simulink model "TopLevelModel"  (R2023a)
settings: Solver=VariableStepAuto  StartTime=0.0  StopTime=inf  RelTol=1e-3
values from neighbouring files (symbols this model uses):
  b = 40.6518    [TopLevelModelParameters.m]
  B1 = 0.0042    [TopLevelModelParameters.m]
  B2 = 0.0084    [TopLevelModelParameters.m]
  J1 = 7e-5    (= 7e-05)    [TopLevelModelParameters.m]
  J2 = 8e-5    (= 8e-05)    [TopLevelModelParameters.m]
  k1 = 2.6552e5    (= 265520)    [TopLevelModelParameters.m]
  k2 = 2.6552e5    (= 265520)    [TopLevelModelParameters.m]
  k3 = 11.777e4    (= 117770)    [TopLevelModelParameters.m]
  Kb = 23e-3    (= 0.023)    [TopLevelModelParameters.m]
  Kt = 23e-3    (= 0.023)    [TopLevelModelParameters.m]
  L = 0.1    [TopLevelModelParameters.m]
  m = 2    [TopLevelModelParameters.m]
  R = 0.71    [TopLevelModelParameters.m]
  r = 0.0194    [TopLevelModelParameters.m]
undefined symbols (not defined in the file or in its folder): J, Kd, Ke
libraries: fl_lib x40, fl_ps_legacy_lib x16, nesl_utility x12, slpidlib x10, SignalEditorBlockLib x4, ee_lib x4, simulink x2
(part 1 of 3)
settings Model: PacingRate=10  Creator=M3tal  LastModifiedBy=M3tal
settings OptimizationCC: DefaultParameterBehavior=Inlined  EnhancedBackFolding=on  PassReuseOutputArgsThreshold=0  OptimizeBlockOrder=speed  DifferentSizesBufferReuse=on
settings DebuggingCC: ParameterTunabilityLossMsg=error
settings HardwareCC: TargetBitPerPointer=64  TargetBitPerSizeT=64  TargetBitPerPtrDiffT=64  TargetLongLongMode=on  TargetIntDivRoundTo=Zero  TargetEndianess=LittleEndian  TargetWordSize=64  TargetHWDeviceType=MATLAB Host  ProdEqTarget=off
settings SFSimCC: MATLABDynamicMemAlloc=off
settings RTWCC: GenCodeOnly=on
settings CodeAppCC: ForceParamTrailComments=on  OperatorAnnotations=on
settings ConfigComp: PLC_TargetIDE=codesys23  PLC_MultiTBSigbuilderTimeRange=off  PLC_FoldFBCallOutputVar=off  PLC_RemoveUnusedSSMethodCallArguments=off  PLC_UseCallOutputArgSyntax=off  PLC_EnableUnsignedAndDoubleTypes=off  PLC_EnableUDTSplitting=off  PLC_MaxFieldsInUDT=500  PLC_InlineEnumCastFunction=off

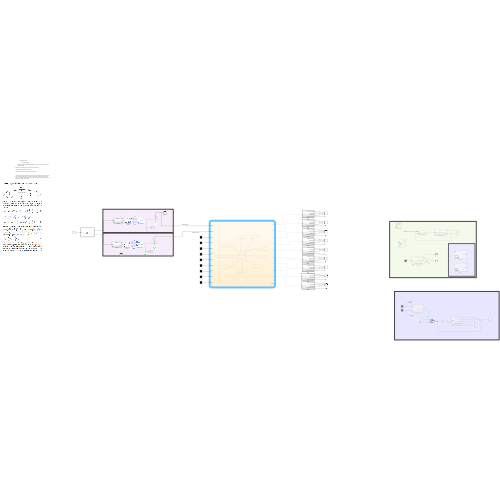
[thumbnail: Simulink's stored preview of the top-level diagram]
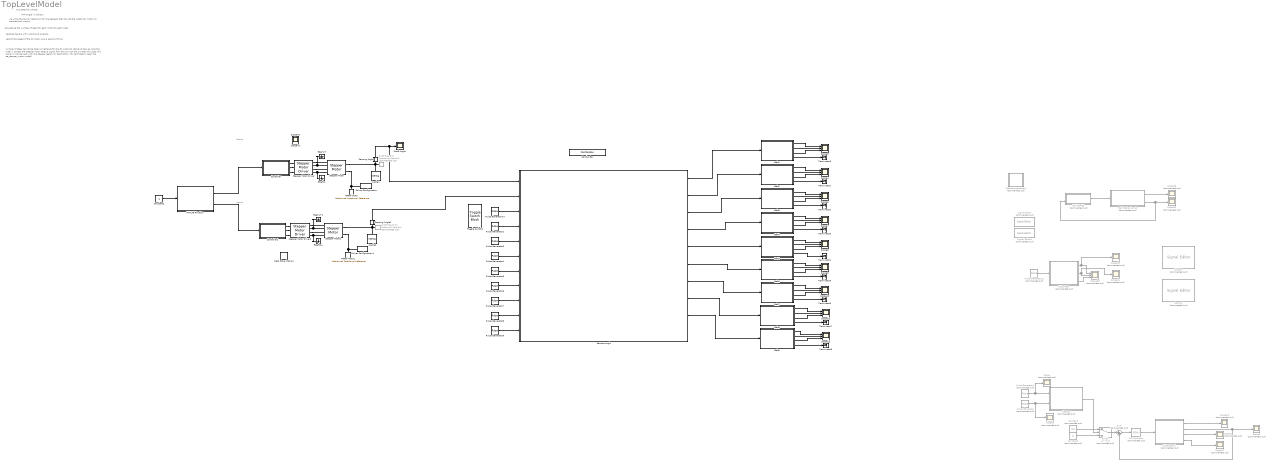
== system TopLevelModel ==
  note: two state flow charts
  note: number of steps cannot be taken as refrence for the dc motors to start and stop as once the meal is chosen the stepper motor takes a signal from the plc with the number of pulses, this signal is maintained unitll the stepper reachs it's destination. (for calrification open the ee_stepper_motor model)
  note: X-axis
  note: -replace signals with inports and outports
  note: -record the speed of the dc motor over a period of time
  note: -caluclating the number of steps for each motor for each meal
  note: Y-axis
  note: we using the same mechansim for the steppers that convert the rotational motion to translational motion
  note: m=r*angle in radians
  Belt Mechanism10 : Subsystem  Commented=on
  Belt1 : Subsystem  TreatAsAtomicUnit=on
  Belt2 : Subsystem  TreatAsAtomicUnit=on
  Belt3 : Subsystem  TreatAsAtomicUnit=on
  Belt4 : Subsystem  TreatAsAtomicUnit=on
  Belt5 : Subsystem  TreatAsAtomicUnit=on
  Belt6 : Subsystem  TreatAsAtomicUnit=on
  Belt7 : Subsystem  TreatAsAtomicUnit=on
  Belt8 : Subsystem  TreatAsAtomicUnit=on
  Belt9 : Subsystem  TreatAsAtomicUnit=on
  Combo Box : ComboBox  LabelPosition=Hide  SelectedLabel=1
      settings: Values={{'1', '2', '3', '4', '5', '6', '7', '8', '9', '0'}, [1 2 3 4 5 6 7 8 9 0]}
  Constant : Constant  Commented=on  Value=0.2
  Constant1 : Constant  Commented=on  Value=0
  Constant2 : Constant
  Controller : Subsystem  Variant=on  VariantControlMode=label  LabelModeActiveChoice=Position
      settings: AttributesFormatString=%<BlockChoice>
  Controller1 : Subsystem  Variant=on  VariantControlMode=label  LabelModeActiveChoice=Position
      settings: AttributesFormatString=%<BlockChoice>
  DC Motor10 : Subsystem  Commented=on
  Data Store Memory : DataStoreMemory  DataStoreName=counter  WriteAfterWriteMsg=warning  ShowAdditionalParam=off
  ERef A+ : fl_lib/Electrical/Electrical Elements/Electrical Reference
  ERef A+1 : fl_lib/Electrical/Electrical Elements/Electrical Reference
  ERef B- : fl_lib/Electrical/Electrical Elements/Electrical Reference
  ERef B-1 : fl_lib/Electrical/Electrical Elements/Electrical Reference
  Inertia1 : fl_lib/Mechanical/Rotational Elements/Inertia  inertia=0.1 kg*m^2  num_ports=foundation.enum.numPorts2.one  w_specify=off  w_priority=High  w=0 rad/s  w_nominal_specify=off  w_nominal_unit=rad/s  w_nominal_value=1  t_specify=off  t_priority=None  t=0 N*m  t_nominal_specify=off  t_nominal_unit=N*m  t_nominal_value=1
  Inertia2 : fl_lib/Mechanical/Rotational Elements/Inertia  inertia=0.1 kg*m^2  num_ports=foundation.enum.numPorts2.one  w_specify=off  w_priority=High  w=0 rad/s  w_nominal_specify=off  w_nominal_unit=rad/s  w_nominal_value=1  t_specify=off  t_priority=None  t=0 N*m  t_nominal_specify=off  t_nominal_unit=N*m  t_nominal_value=1
  MATLAB Function : MATLAB Function  TreatAsAtomicUnit=on
  MRRef Motor : fl_lib/Mechanical/Rotational Elements/Mechanical Rotational Reference
  MRRef Motor1 : fl_lib/Mechanical/Rotational Elements/Mechanical Rotational Reference
  PID Controller : slpidlib/PID Controller  Commented=on  Controller=PID  Form=Parallel  TimeDomain=Continuous-time  UseExternalTs=off  SampleTime=-1  IntegratorMethod=Forward Euler  FilterMethod=Forward Euler  ControllerParametersSource=internal  P=29.8496571480823  I=152.933850283855  UseKiTs=off  D=-0.451147774638306  N=4.48716691500189  UseFilter=on  TunerSelectOption=Transfer Function Based (PID Tuner App)  InitialConditionSource=internal  InitialConditionForIntegrator=0  InitialConditionForFilter=0  DifferentiatorICPrevScaledInput=0  ExternalReset=none  TrackingMode=off  Kt=1  LimitOutput=off  SatLimitsSource=internal  UpperSaturationLimit=inf  LowerSaturationLimit=-inf  LinearizeAsGain=on  AntiWindupMode=none  Kb=1  LimitIntegrator=off  UpperIntegratorSaturationLimit=inf  LowerIntegratorSaturationLimit=-inf  POutMin=[]  POutMax=[]  IOutMin=[]  IOutMax=[]  DOutMin=[]  DOutMax=[]  NOutMin=[]  NOutMax=[]  SumOutMin=[]  SumOutMax=[]  SaturationOutMin=[]  SaturationOutMax=[]  PParamMin=[]  PParamMax=[]  IParamMin=[]  IParamMax=[]  DParamMin=[]  DParamMax=[]  NParamMin=[]  NParamMax=[]  KbParamMin=[]  KbParamMax=[]  KtParamMin=[]  KtParamMax=[]  KbOutMin=[]  KbOutMax=[]  KtOutMin=[]  KtOutMax=[]  IntegratorOutMin=[]  IntegratorOutMax=[]  FilterOutMin=[]  FilterOutMax=[]  SumI1OutMin=[]  SumI1OutMax=[]  SumI2OutMin=[]  SumI2OutMax=[]  SumI3OutMin=[]  SumI3OutMax=[]  SumI4OutMin=[]  SumI4OutMax=[]  SumDOutMin=[]  SumDOutMax=[]  DifferentiatorOutMin=[]  DifferentiatorOutMax=[]  FilterDiffOutCoefMin=[]  FilterDiffOutCoefMax=[]  ReciprocalOutMin=[]  ReciprocalOutMax=[]  SumDenOutMin=[]  SumDenOutMax=[]  SumNumOutMin=[]  SumNumOutMax=[]  DivideOutMin=[]  DivideOutMax=[]  UdiffTsProdOutMin=[]  UdiffTsProdOutMax=[]  NTsProdOutMin=[]  NTsProdOutMax=[]  UintegralTsProdOutMin=[]  UintegralTsProdOutMax=[]  UngainTsProdOutMin=[]  UngainTsProdOutMax=[]  ClampingZeroOutDataTypeStr=Inherit: Inherit via back propagation  ClampingZeroOutMin=[]  ClampingZeroOutMax=[]  FilterDenConstantOutDataTypeStr=Inherit: Inherit via back propagation  FilterDenConstantOutMin=[]  FilterDenConstantOutMax=[]  PCopyOutDataTypeStr=Inherit: Inherit via back propagation  PCopyOutMin=[]  PCopyOutMax=[]  NCopyOutDataTypeStr=Inherit: Inherit via back propagation  NCopyOutMin=[]  NCopyOutMax=[]  IntegratorContinuousStateAttributes=''  IntegratorStateMustResolveToSignalObject=off  IntegratorRTWStateStorageClass=Auto  FilterContinuousStateAttributes=''  FilterStateMustResolveToSignalObject=off  FilterRTWStateStorageClass=Auto  ParallelPVariant=InternalParameters  IdealPVariant=Disabled  IVariant=InternalParameters  DVariant=InternalParameters  IntegratorVariant=Continuous  SatVariant=Disabled  AWVariant=Passthrough  PCopyVariant=Disabled  TRVariant=Disabled  FdbkBlocksVariant=Forward  IdealPFdbkVariant=Disabled  SatFdbkVariant=Disabled  DerivativeFilterVariant=ContFilter  NVariant=InternalParameters  NCopyVariant=Disabled  FilterICVariant=InternalICsFilter  IntegratorICVariant=InternalICs  ExternalResetVariant=Disabled  TRSumVariant=Passthrough  SumFdbkVariant=Disabled  SumVariant=Sum_PID  TsampFilterVariant=InternalTs  TsampNgainVariant=Passthrough  TsampIntegralVariant=Disabled_SignalSpec  ExternalSaturationOutDataTypeStr=Inherit: Same as second input
  Pulse Generator : DiscretePulseGenerator  Commented=on  PulseType=Time based  Period=40  PhaseDelay=20
  Pulse Generator1 : DiscretePulseGenerator  Commented=on  PulseType=Time based  Period=50  PhaseDelay=5
  Pulse Generator11 : DiscretePulseGenerator  Commented=on  PulseType=Time based  Amplitude=12  Period=11  PulseWidth=50  PhaseDelay=2
  Pulse Generator14 : DiscretePulseGenerator  PulseType=Time based  Period=10  PulseWidth=5
  Pulse Generator{2..9} (8 alike) : DiscretePulseGenerator  PulseType=Time based  Amplitude=0  Period=10  PulseWidth=5
  Scope{,1..3,24..29} (10 alike) : Scope  Commented=on
  Scope{4..12} (9 alike) : Scope  NumInputPorts=3
  Scope23 : Scope  Commented=on  NumInputPorts=3
  Sensing Angle : Subsystem
      mask Display: disp('a')
  Sensing Angle1 : Subsystem
      mask Display: disp('a')
  Sensor : SignalEditorBlockLib/Signal Editor  Commented=on  FileName=Crane_Sensor.mat  ActiveScenario=Scenario  ActiveSignal=Crane signal  IsBus=off  OutputBusObjectStr=Bus: BusObject  SampleTime=0  Interpolate=off  ZeroCross=off  OutputAfterFinalValue=Setting to zero  Unit=inherit  PreserveSignalName=on  ApplySigPropsToAllScenarios=on
  Sensor1 : SignalEditorBlockLib/Signal Editor  Commented=on  FileName=Belt_Sensor.mat  ActiveScenario=Scenario  ActiveSignal=Belt Signal  IsBus=off  OutputBusObjectStr=Bus: BusObject  SampleTime=0  Interpolate=off  ZeroCross=off  OutputAfterFinalValue=Setting to zero  Unit=inherit  PreserveSignalName=on  ApplySigPropsToAllScenarios=on
  Sensors : Stateflow chart  Commented=on  TreatAsAtomicUnit=on
  Sensors Logic : Stateflow chart  TreatAsAtomicUnit=on
      settings: PortSchema="{\"entries\":[{\"content\":{\"sides\":[{\"content\":{\"connectorIds\":[\"In10\",\"In11\",\"In1\",\"In2\",\"In3\",\"In4\",\"In5\",\"In6\",\"In7\",\"In8\",\"In9\"]},\"type\":\"ConnectorPlacement.EquallySpacedRectSide\",\"uuid\":\"dd9ce701-3689-4654-9b21-5529dab0541a\"},{\"content\":{\"connectorIds\":[\"Out1\",\"Out2\",\"Out3\",\"Out4\",\"Out5\",\"Out6\",\"Out7\",\"Out8\",\"Out9\",\"Out10\"],\"side\":\"RIGHT\"},\"type\":\"ConnectorPlacement.EquallySpacedRectSide\",\"uuid\":\"ff8f0f67-846c-4703-aeda-d87216d47c92\"},{\"content\":{\"side\":\"TOP\"},\"type\":\"ConnectorPlacement.EquallySpacedRectSide\",\"uuid\":\"ae968bb7-da0f-44fd-802b-06f57922bbce\"},{\"content\":{\"side\":\"BOTTOM\"},\"type\":\"ConnectorPlacement.EquallySpacedRectSide\",\"uuid\":\"72f2caf6-56e4-41be-9339-a06e52f77ea7\"}]},\"type\":\"ConnectorPlacement.EquallySpacedConnector\",\"uuid\":\"820653e5-881f-4b8b-9810-894dc5dde637\"}],\"packageUris\":[\"http://schema.mathworks.com/mf0/Connector/R2020b\"],\"version\":\"1.0\"}"
  Shaft Angle : Scope
  Shaft Free End : fl_lib/Mechanical/Rotational Elements/Rotational Free End  Commented=on  w_specify=off  w_priority=None  w=0 rad/s  w_nominal_specify=off  w_nominal_unit=rad/s  w_nominal_value=1
  Shaft Free End1 : fl_lib/Mechanical/Rotational Elements/Rotational Free End  Commented=on  w_specify=off  w_priority=None  w=0 rad/s  w_nominal_specify=off  w_nominal_unit=rad/s  w_nominal_value=1
  Signal Editor : SignalEditorBlockLib/Signal Editor  Commented=on  FileName=X_Position.mat  ActiveScenario=Scenario  ActiveSignal=X  IsBus=off  OutputBusObjectStr=Bus: BusObject  SampleTime=0  Interpolate=off  ZeroCross=off  OutputAfterFinalValue=Setting to zero  Unit=inherit  PreserveSignalName=on  ApplySigPropsToAllScenarios=on
  Signal Editor1 : SignalEditorBlockLib/Signal Editor  Commented=on  FileName=Y_Position.mat  ActiveScenario=Scenario  ActiveSignal=Y  IsBus=off  OutputBusObjectStr=Bus: BusObject  SampleTime=0  Interpolate=off  ZeroCross=off  OutputAfterFinalValue=Setting to zero  Unit=inherit  PreserveSignalName=on  ApplySigPropsToAllScenarios=on
  Solver Configuration : nesl_utility/Solver Configuration  PhysicalDomain=network_engine_domain  SubClassName=solver  LeftPortType=input  RightPortType=generic  Tones=[]  Harmonics=[]  SimulateNoise=off  Profile=off  UseLocalSampling=off  EnableSwitchedLinearOptims=on  FrequencyDomain=off  UseCCode=off  RelTol=0.001  AbsTol=1e-06  MinStep=1e-09  ToWorkspace=off  RevertToSquareIcSolve=off  NumHomotopyIterations=100  PhasorMode=off  PhasorModeNumHarmonics=1  ConsistencySolver=NEWTON_FTOL  IndexReductionMethod=DerivativeReplacement  DoDC=off  ResidualTolerance=1e-9  ConsistencyTolSource=GLOBAL  ConsistencyAbsTol=0.001  ConsistencyRelTol=0.001  ConsistencyTolFactor=0.001  UseLocalSolver=off  LocalSolverChoice=NE_BACKWARD_EULER_ADVANCER  ResolveIndetEquations=on  FunctionEvalNumThread=1  LocalSolverSampleTime=.001  DoFixedCost=off  MaxNonlinIter=3  MaxModeIter=2  ComputeImpulses=off  ImpulseIterations=2  LinearAlgebra=auto  LinearAlgebraNumThread=0  EquationFormulation=NE_TIME_EF  DelaysMemoryBudget=1024  AutomaticFiltering=on  FilteringTimeConstant=0.001  PartitionStorageMethod=AS_NEEDED  PartitionMemoryBudget=1024  PartitionMethod=FAST
  Solver Configuration1 : nesl_utility/Solver Configuration  PhysicalDomain=network_engine_domain  SubClassName=solver  LeftPortType=input  RightPortType=generic  Tones=[]  Harmonics=[]  SimulateNoise=off  Profile=off  UseLocalSampling=off  EnableSwitchedLinearOptims=on  FrequencyDomain=off  UseCCode=off  RelTol=0.001  AbsTol=1e-06  MinStep=1e-09  ToWorkspace=off  RevertToSquareIcSolve=off  NumHomotopyIterations=100  PhasorMode=off  PhasorModeNumHarmonics=1  ConsistencySolver=NEWTON_FTOL  IndexReductionMethod=DerivativeReplacement  DoDC=off  ResidualTolerance=1e-9  ConsistencyTolSource=GLOBAL  ConsistencyAbsTol=0.001  ConsistencyRelTol=0.001  ConsistencyTolFactor=0.001  UseLocalSolver=off  LocalSolverChoice=NE_BACKWARD_EULER_ADVANCER  ResolveIndetEquations=on  FunctionEvalNumThread=1  LocalSolverSampleTime=.001  DoFixedCost=off  MaxNonlinIter=3  MaxModeIter=2  ComputeImpulses=off  ImpulseIterations=2  LinearAlgebra=auto  LinearAlgebraNumThread=0  EquationFormulation=NE_TIME_EF  DelaysMemoryBudget=1024  AutomaticFiltering=on  FilteringTimeConstant=0.001  PartitionStorageMethod=AS_NEEDED  PartitionMemoryBudget=1024  PartitionMethod=FAST
  Stepper Motor : ee_lib/Electromechanical/Reluctance & Stepper/Stepper Motor  step_or_av=ee.enum.electromech.simulationMode.stepping  Ra=1.3 Ohm  La=2.9 mH  Km=0.315 N*m/A  Td=25 mN*m  Rm=Inf Ohm  w_vec=[ 0 1000 3e+3 ] rpm  T_vec=[ 2 2 1 ] N*m  assert_if_slipping=0  J_total=1e-4 kg*m^2  max_step_rate=10 Hz  Step=1.8 deg  J=82 g*cm^2  B=1e-2 N*m/(rad/s)  speed0=0 rpm  theta0=0 deg  alpha=[.00393, .00393] 1/K  Tmeas=25 degC  Tmeas2=125 degC  T_vec2=[1.7, 1.7, .85] N*m  half_stepping=ee.enum.electromech.steppingModeAveraged.fullStep  thermal_masses=[100, 100] J/K  initial_temperatures=[25, 25] degC  rotor_thermal_mass=50 J/K  rotor_initial_temperature=25 degC  Rm_percent_rotor=90
      settings: InternalSimscapePortConfiguration="{\"Bottom\":[],\"Left\":[{\"id\":\"pA\",\"label\":\"A+\",\"type\":\"foundation.electrical.electrical\"},{\"id\":\"nA\",\"label\":\"A-\",\"type\":\"foundation.electrical.electrical\"},{\"id\":\"pB\",\"label\":\"B+\",\"type\":\"foundation.electrical.electrical\"},{\"id\":\"nB\",\"label\":\"B-\",\"type\":\"foundation.electrical.electrical\"}],\"Right\":[{\"id\":\"R\",\"label\":\"R\",\"type\":\"foundation.mechanical.rotational.rotational\"},{\"id\":\"C\",\"label\":\"C\",\"type\":\"foundation.mechanical.rotational.rotational\"}],\"Top\":[]}"
  Stepper Motor Driver : ee_lib/Electromechanical/Reluctance & Stepper/Stepper Motor Driver  step_or_av=1  step_rate_per_volt=10 Hz/V  Venable=2.5 V  Vreverse=2.5 V  supply_ports=ee.enum.supply_ports.hidesupply  Vm=5 V  Vsupply=10 V  half_stepping=0  stepping_mode=ee.enum.electromech.steppingMode.fullStep  numMicroSteps=4  Im=1.2 A
      settings: InternalSimscapePortConfiguration="{\"Bottom\":[],\"Left\":[{\"id\":\"ENA\",\"label\":\"ENA\",\"type\":\"foundation.electrical.electrical\"},{\"id\":\"REF\",\"label\":\"REF\",\"type\":\"foundation.electrical.electrical\"},{\"id\":\"REV\",\"label\":\"REV\",\"type\":\"foundation.electrical.electrical\"}],\"Right\":[{\"id\":\"pA\",\"label\":\"A+\",\"type\":\"foundation.electrical.electrical\"},{\"id\":\"nA\",\"label\":\"A-\",\"type\":\"foundation.electrical.electrical\"},{\"id\":\"pB\",\"label\":\"B+\",\"type\":\"foundation.electrical.electrical\"},{\"id\":\"nB\",\"label\":\"B-\",\"type\":\"foundation.electrical.electrical\"}],\"Top\":[]}"
  Stepper Motor Driver1 : ee_lib/Electromechanical/Reluctance & Stepper/Stepper Motor Driver  step_or_av=1  step_rate_per_volt=10 Hz/V  Venable=2.5 V  Vreverse=2.5 V  supply_ports=ee.enum.supply_ports.hidesupply  Vm=5 V  Vsupply=10 V  half_stepping=0  stepping_mode=ee.enum.electromech.steppingMode.fullStep  numMicroSteps=4  Im=1.2 A
      settings: InternalSimscapePortConfiguration="{\"Bottom\":[],\"Left\":[{\"id\":\"ENA\",\"label\":\"ENA\",\"type\":\"foundation.electrical.electrical\"},{\"id\":\"REF\",\"label\":\"REF\",\"type\":\"foundation.electrical.electrical\"},{\"id\":\"REV\",\"label\":\"REV\",\"type\":\"foundation.electrical.electrical\"}],\"Right\":[{\"id\":\"pA\",\"label\":\"A+\",\"type\":\"foundation.electrical.electrical\"},{\"id\":\"nA\",\"label\":\"A-\",\"type\":\"foundation.electrical.electrical\"},{\"id\":\"pB\",\"label\":\"B+\",\"type\":\"foundation.electrical.electrical\"},{\"id\":\"nB\",\"label\":\"B-\",\"type\":\"foundation.electrical.electrical\"}],\"Top\":[]}"
  Stepper Motor1 : ee_lib/Electromechanical/Reluctance & Stepper/Stepper Motor  step_or_av=ee.enum.electromech.simulationMode.stepping  Ra=1.3 Ohm  La=2.9 mH  Km=0.315 N*m/A  Td=25 mN*m  Rm=Inf Ohm  w_vec=[ 0 1000 3e+3 ] rpm  T_vec=[ 2 2 1 ] N*m  assert_if_slipping=0  J_total=1e-4 kg*m^2  max_step_rate=10 Hz  Step=1.8 deg  J=82 g*cm^2  B=1e-2 N*m/(rad/s)  speed0=0 rpm  theta0=0 deg  alpha=[.00393, .00393] 1/K  Tmeas=25 degC  Tmeas2=125 degC  T_vec2=[1.7, 1.7, .85] N*m  half_stepping=ee.enum.electromech.steppingModeAveraged.fullStep  thermal_masses=[100, 100] J/K  initial_temperatures=[25, 25] degC  rotor_thermal_mass=50 J/K  rotor_initial_temperature=25 degC  Rm_percent_rotor=90
      settings: InternalSimscapePortConfiguration="{\"Bottom\":[],\"Left\":[{\"id\":\"pA\",\"label\":\"A+\",\"type\":\"foundation.electrical.electrical\"},{\"id\":\"nA\",\"label\":\"A-\",\"type\":\"foundation.electrical.electrical\"},{\"id\":\"pB\",\"label\":\"B+\",\"type\":\"foundation.electrical.electrical\"},{\"id\":\"nB\",\"label\":\"B-\",\"type\":\"foundation.electrical.electrical\"}],\"Right\":[{\"id\":\"R\",\"label\":\"R\",\"type\":\"foundation.mechanical.rotational.rotational\"},{\"id\":\"C\",\"label\":\"C\",\"type\":\"foundation.mechanical.rotational.rotational\"}],\"Top\":[]}"
  SteppermotorsLogic : Stateflow chart  Commented=on  TreatAsAtomicUnit=on
  Subsystem : Subsystem  Commented=on
  Subsystem1 : Subsystem  Commented=on
  Sum : Sum  Commented=on  Inputs=|+-
  Switch : Switch  Commented=on  Criteria=u2 ~= 0  Threshold=1  SaturateOnIntegerOverflow=off  InputSameDT=off
  Terminator{1..9} (9 alike) : Terminator
  Toggle Switch2 : ToggleSwitchBlock
      settings: Values={{'Off', 'On'}, [0 1]}
  Scope41 : Scope
  Scope42 : Scope
  wires:
  Pulse Generator1/1 -> Scope/1, Sensors/1(Crane)
  Subsystem1/2(load velocity) -> Sum/2, Scope2/1  "Velocity"
  Pulse Generator/1 -> Scope3/1, Sensors/2(Belt)
  Subsystem/1(drive pulley velocity) -> Scope25/1, Scope23/1
  Subsystem/2(load velocity) -> Scope23/2, Scope24/1
  Subsystem/3(driven pulley velocity) -> Scope23/3
  Pulse Generator11/1 -> Subsystem/1(Voltage)
  Sum/1 -> PID Controller/1
  Sensors/1(Voltage) -> Switch/2
  Constant1/1 -> Switch/3
  PID Controller/1 -> Subsystem1/1(Voltage)
  Switch/1 -> Sum/1
  Constant/1 -> Switch/1
  Subsystem1/1(drive pulley velocity) -> Scope26/1
  Subsystem1/4(driven pulley Velocity) -> Scope27/1
  Subsystem1/3(load position) -> Scope1/1
  Constant2/1 -> MATLAB Function/1(meal)
  ? -> DC Motor10/1(Voltage)
  Belt Mechanism10/2(Velocity) -> Scope29/1, DC Motor10/2(Velocity)  "Velocity"
  Belt Mechanism10/1(Position) -> Scope28/1
  DC Motor10/1(Tourque) -> Belt Mechanism10/1(Tourque)  "Tourque"
  Sensing Angle/1(theta) -> Sensors Logic/10(XTheta), Shaft Angle/1  "XTheta (degrees)"
  Sensing Angle1/1(theta) -> Sensors Logic/11(YTheta)  "YTheta (degrees)"
  MATLAB Function/1(x) -> Controller/1(Ref)
  Pulse Generator14/1 -> Sensors Logic/1(Belt1)
  MATLAB Function/2(y) -> Controller1/1(Ref)
  Sensors Logic/1(V1) -> Belt1/1(V1)
  Belt1/4(driven pulley Velocity) -> Terminator9/1
  Belt1/1(drive pulley velocity) -> Scope5/1
  Belt1/2(load velocity) -> Scope5/2
  Belt1/3(load position) -> Scope5/3
  Belt2/1(drive pulley velocity) -> Scope4/1
  Belt2/3(load position) -> Scope4/3
  Belt2/4(driven pulley Velocity) -> Terminator1/1
  Belt2/2(load velocity) -> Scope4/2
  Sensors Logic/2(V2) -> Belt2/1(V1)
  Belt3/2(load velocity) -> Scope6/2
  Belt3/1(drive pulley velocity) -> Scope6/1
  Belt3/3(load position) -> Scope6/3
  Belt3/4(driven pulley Velocity) -> Terminator2/1
  Sensors Logic/3(V3) -> Belt3/1(V1)
  Belt4/4(driven pulley Velocity) -> Terminator3/1
  Belt4/3(load position) -> Scope7/3
  Belt4/2(load velocity) -> Scope7/2
  Belt4/1(drive pulley velocity) -> Scope7/1
  Sensors Logic/4(V4) -> Belt4/1(V1)
  Sensors Logic/5(V5) -> Belt5/1(V1)
  Belt5/3(load position) -> Scope8/3
  Belt5/1(drive pulley velocity) -> Scope8/1
  Belt5/4(driven pulley Velocity) -> Terminator4/1
  Belt5/2(load velocity) -> Scope8/2
  Belt6/2(load velocity) -> Scope9/2
  Belt6/4(driven pulley Velocity) -> Terminator5/1
  Belt6/3(load position) -> Scope9/3
  Belt6/1(drive pulley velocity) -> Scope9/1
  Sensors Logic/6(V6) -> Belt6/1(V1)
  Belt7/3(load position) -> Scope10/3
  Belt7/1(drive pulley velocity) -> Scope10/1
  Belt7/2(load velocity) -> Scope10/2
  Belt7/4(driven pulley Velocity) -> Terminator6/1
  Sensors Logic/7(V7) -> Belt7/1(V1)
  Belt8/1(drive pulley velocity) -> Scope11/1
  Belt8/3(load position) -> Scope11/3
  Belt8/4(driven pulley Velocity) -> Terminator7/1
  Belt8/2(load velocity) -> Scope11/2
  Sensors Logic/8(V8) -> Belt8/1(V1)
  Belt9/3(load position) -> Scope12/3
  Belt9/2(load velocity) -> Scope12/2
  Belt9/4(driven pulley Velocity) -> Terminator8/1
  Belt9/1(drive pulley velocity) -> Scope12/1
  Sensors Logic/9(V9) -> Belt9/1(V1)
  Pulse Generator2/1 -> Sensors Logic/2(Belt2)
  Pulse Generator4/1 -> Sensors Logic/4(Belt4)
  Pulse Generator3/1 -> Sensors Logic/3(Belt3)
  Pulse Generator5/1 -> Sensors Logic/5(Belt5)
  Pulse Generator6/1 -> Sensors Logic/6(Belt6)
  Pulse Generator7/1 -> Sensors Logic/7(Belt7)
  Pulse Generator8/1 -> Sensors Logic/8(Belt8)
  Pulse Generator9/1 -> Sensors Logic/9(Belt9)
  connections:
  MRRef Motor/LConn1 -- Stepper Motor/RConn2 -- Solver Configuration/RConn1
  Stepper Motor/LConn4 -- Stepper Motor Driver/RConn4 -- ERef B-/LConn1
  Stepper Motor Driver/RConn2 -- Stepper Motor/LConn2 -- ERef A+/LConn1
  Sensing Angle/LConn1 -- Stepper Motor/RConn1 -- Inertia1/LConn1 -- Shaft Free End/LConn1
  Stepper Motor Driver/RConn1 -- Stepper Motor/LConn1
  Controller/RConn2 -- Stepper Motor Driver/LConn2
  Controller/RConn3 -- Stepper Motor Driver/LConn3
  Controller/RConn1 -- Stepper Motor Driver/LConn1
  Stepper Motor Driver/RConn3 -- Stepper Motor/LConn3
  ERef B-1/LConn1 -- Stepper Motor1/LConn4 -- Stepper Motor Driver1/RConn4
  Solver Configuration1/RConn1 -- MRRef Motor1/LConn1 -- Stepper Motor1/RConn2
  ERef A+1/LConn1 -- Stepper Motor Driver1/RConn2 -- Stepper Motor1/LConn2
  Sensing Angle1/LConn1 -- Stepper Motor1/RConn1 -- Inertia2/LConn1 -- Shaft Free End1/LConn1
  Controller1/RConn3 -- Stepper Motor Driver1/LConn3
  Controller1/RConn1 -- Stepper Motor Driver1/LConn1
  Stepper Motor Driver1/RConn1 -- Stepper Motor1/LConn1
  Stepper Motor Driver1/RConn3 -- Stepper Motor1/LConn3
  Controller1/RConn2 -- Stepper Motor Driver1/LConn2

== system TopLevelModel/Belt Mechanism10 ==
  note: Note: The term $K \frac{d\theta}{dt}$ ​ represents a damping torque that is proportional to the angular velocity
  note: $\frac{d^2\theta}{dt^2} = \frac{1}{J} \left(T - K \frac{d\theta}{dt}\right)$
      | belt mechanism equaition based on newton seconed law for rotational motion
  Tourque : Inport
  Gain1 : Gain  Gain=1/J
  Integrator2 : Integrator
  Integrator3 : Integrator
  Subtract : Sum  Inputs=+-
  damping coefficient : Gain  Gain=Kd
  Position : Outport
  Velocity : Outport  Port=2
  wires:
  Integrator2/1 -> damping coefficient/1, Velocity/1, Integrator3/1  "Velocity"
  Tourque/1 -> Subtract/1
  Subtract/1 -> Gain1/1
  Integrator3/1 -> Position/1  "Position"
  damping coefficient/1 -> Subtract/2
  Gain1/1 -> Integrator2/1  "theta_dot_dot"

== system TopLevelModel/Belt1 ==
  V1 : Inport
  Constant3 : Constant  Value=0.2
  Constant4 : Constant  Value=0
  PID Controller1 : slpidlib/PID Controller  Controller=PID  Form=Parallel  TimeDomain=Continuous-time  UseExternalTs=off  SampleTime=-1  IntegratorMethod=Forward Euler  FilterMethod=Forward Euler  ControllerParametersSource=internal  P=29.8496571480823  I=152.933850283855  UseKiTs=off  D=-0.451147774638306  N=4.48716691500189  UseFilter=on  TunerSelectOption=Transfer Function Based (PID Tuner App)  InitialConditionSource=internal  InitialConditionForIntegrator=0  InitialConditionForFilter=0  DifferentiatorICPrevScaledInput=0  ExternalReset=none  TrackingMode=off  Kt=1  LimitOutput=off  SatLimitsSource=internal  UpperSaturationLimit=inf  LowerSaturationLimit=-inf  LinearizeAsGain=on  AntiWindupMode=none  Kb=1  LimitIntegrator=off  UpperIntegratorSaturationLimit=inf  LowerIntegratorSaturationLimit=-inf  POutMin=[]  POutMax=[]  IOutMin=[]  IOutMax=[]  DOutMin=[]  DOutMax=[]  NOutMin=[]  NOutMax=[]  SumOutMin=[]  SumOutMax=[]  SaturationOutMin=[]  SaturationOutMax=[]  PParamMin=[]  PParamMax=[]  IParamMin=[]  IParamMax=[]  DParamMin=[]  DParamMax=[]  NParamMin=[]  NParamMax=[]  KbParamMin=[]  KbParamMax=[]  KtParamMin=[]  KtParamMax=[]  KbOutMin=[]  KbOutMax=[]  KtOutMin=[]  KtOutMax=[]  IntegratorOutMin=[]  IntegratorOutMax=[]  FilterOutMin=[]  FilterOutMax=[]  SumI1OutMin=[]  SumI1OutMax=[]  SumI2OutMin=[]  SumI2OutMax=[]  SumI3OutMin=[]  SumI3OutMax=[]  SumI4OutMin=[]  SumI4OutMax=[]  SumDOutMin=[]  SumDOutMax=[]  DifferentiatorOutMin=[]  DifferentiatorOutMax=[]  FilterDiffOutCoefMin=[]  FilterDiffOutCoefMax=[]  ReciprocalOutMin=[]  ReciprocalOutMax=[]  SumDenOutMin=[]  SumDenOutMax=[]  SumNumOutMin=[]  SumNumOutMax=[]  DivideOutMin=[]  DivideOutMax=[]  UdiffTsProdOutMin=[]  UdiffTsProdOutMax=[]  NTsProdOutMin=[]  NTsProdOutMax=[]  UintegralTsProdOutMin=[]  UintegralTsProdOutMax=[]  UngainTsProdOutMin=[]  UngainTsProdOutMax=[]  ClampingZeroOutDataTypeStr=Inherit: Inherit via back propagation  ClampingZeroOutMin=[]  ClampingZeroOutMax=[]  FilterDenConstantOutDataTypeStr=Inherit: Inherit via back propagation  FilterDenConstantOutMin=[]  FilterDenConstantOutMax=[]  PCopyOutDataTypeStr=Inherit: Inherit via back propagation  PCopyOutMin=[]  PCopyOutMax=[]  NCopyOutDataTypeStr=Inherit: Inherit via back propagation  NCopyOutMin=[]  NCopyOutMax=[]  IntegratorContinuousStateAttributes=''  IntegratorStateMustResolveToSignalObject=off  IntegratorRTWStateStorageClass=Auto  FilterContinuousStateAttributes=''  FilterStateMustResolveToSignalObject=off  FilterRTWStateStorageClass=Auto  ParallelPVariant=InternalParameters  IdealPVariant=Disabled  IVariant=InternalParameters  DVariant=InternalParameters  IntegratorVariant=Continuous  SatVariant=Disabled  AWVariant=Passthrough  PCopyVariant=Disabled  TRVariant=Disabled  FdbkBlocksVariant=Forward  IdealPFdbkVariant=Disabled  SatFdbkVariant=Disabled  DerivativeFilterVariant=ContFilter  NVariant=InternalParameters  NCopyVariant=Disabled  FilterICVariant=InternalICsFilter  IntegratorICVariant=InternalICs  ExternalResetVariant=Disabled  TRSumVariant=Passthrough  SumFdbkVariant=Disabled  SumVariant=Sum_PID  TsampFilterVariant=InternalTs  TsampNgainVariant=Passthrough  TsampIntegralVariant=Disabled_SignalSpec  ExternalSaturationOutDataTypeStr=Inherit: Same as second input
  Subsystem2 : Subsystem
  Sum1 : Sum  Inputs=|+-
  Switch1 : Switch  Criteria=u2 ~= 0  Threshold=1  SaturateOnIntegerOverflow=off  InputSameDT=off
  drive pulley velocity : Outport
  load velocity : Outport  Port=2
  load position : Outport  Port=3
  driven pulley Velocity : Outport  Port=4
  wires:
  Switch1/1 -> Sum1/1
  Sum1/1 -> PID Controller1/1
  V1/1 -> Switch1/2
  Subsystem2/2(load velocity) -> load velocity/1, Sum1/2  "Velocity"
  Constant3/1 -> Switch1/1
  Constant4/1 -> Switch1/3
  PID Controller1/1 -> Subsystem2/1(Voltage)
  Subsystem2/3(load position) -> load position/1
  Subsystem2/4(driven pulley Velocity) -> driven pulley Velocity/1
  Subsystem2/1(drive pulley velocity) -> drive pulley velocity/1

== system TopLevelModel/Belt2 ==
  V1 : Inport
  Constant3 : Constant  Commented=on  Value=0.2
  Constant4 : Constant  Commented=on  Value=0
  PID Controller1 : slpidlib/PID Controller  Commented=on  Controller=PID  Form=Parallel  TimeDomain=Continuous-time  UseExternalTs=off  SampleTime=-1  IntegratorMethod=Forward Euler  FilterMethod=Forward Euler  ControllerParametersSource=internal  P=29.8496571480823  I=152.933850283855  UseKiTs=off  D=-0.451147774638306  N=4.48716691500189  UseFilter=on  TunerSelectOption=Transfer Function Based (PID Tuner App)  InitialConditionSource=internal  InitialConditionForIntegrator=0  InitialConditionForFilter=0  DifferentiatorICPrevScaledInput=0  ExternalReset=none  TrackingMode=off  Kt=1  LimitOutput=off  SatLimitsSource=internal  UpperSaturationLimit=inf  LowerSaturationLimit=-inf  LinearizeAsGain=on  AntiWindupMode=none  Kb=1  LimitIntegrator=off  UpperIntegratorSaturationLimit=inf  LowerIntegratorSaturationLimit=-inf  POutMin=[]  POutMax=[]  IOutMin=[]  IOutMax=[]  DOutMin=[]  DOutMax=[]  NOutMin=[]  NOutMax=[]  SumOutMin=[]  SumOutMax=[]  SaturationOutMin=[]  SaturationOutMax=[]  PParamMin=[]  PParamMax=[]  IParamMin=[]  IParamMax=[]  DParamMin=[]  DParamMax=[]  NParamMin=[]  NParamMax=[]  KbParamMin=[]  KbParamMax=[]  KtParamMin=[]  KtParamMax=[]  KbOutMin=[]  KbOutMax=[]  KtOutMin=[]  KtOutMax=[]  IntegratorOutMin=[]  IntegratorOutMax=[]  FilterOutMin=[]  FilterOutMax=[]  SumI1OutMin=[]  SumI1OutMax=[]  SumI2OutMin=[]  SumI2OutMax=[]  SumI3OutMin=[]  SumI3OutMax=[]  SumI4OutMin=[]  SumI4OutMax=[]  SumDOutMin=[]  SumDOutMax=[]  DifferentiatorOutMin=[]  DifferentiatorOutMax=[]  FilterDiffOutCoefMin=[]  FilterDiffOutCoefMax=[]  ReciprocalOutMin=[]  ReciprocalOutMax=[]  SumDenOutMin=[]  SumDenOutMax=[]  SumNumOutMin=[]  SumNumOutMax=[]  DivideOutMin=[]  DivideOutMax=[]  UdiffTsProdOutMin=[]  UdiffTsProdOutMax=[]  NTsProdOutMin=[]  NTsProdOutMax=[]  UintegralTsProdOutMin=[]  UintegralTsProdOutMax=[]  UngainTsProdOutMin=[]  UngainTsProdOutMax=[]  ClampingZeroOutDataTypeStr=Inherit: Inherit via back propagation  ClampingZeroOutMin=[]  ClampingZeroOutMax=[]  FilterDenConstantOutDataTypeStr=Inherit: Inherit via back propagation  FilterDenConstantOutMin=[]  FilterDenConstantOutMax=[]  PCopyOutDataTypeStr=Inherit: Inherit via back propagation  PCopyOutMin=[]  PCopyOutMax=[]  NCopyOutDataTypeStr=Inherit: Inherit via back propagation  NCopyOutMin=[]  NCopyOutMax=[]  IntegratorContinuousStateAttributes=''  IntegratorStateMustResolveToSignalObject=off  IntegratorRTWStateStorageClass=Auto  FilterContinuousStateAttributes=''  FilterStateMustResolveToSignalObject=off  FilterRTWStateStorageClass=Auto  ParallelPVariant=InternalParameters  IdealPVariant=Disabled  IVariant=InternalParameters  DVariant=InternalParameters  IntegratorVariant=Continuous  SatVariant=Disabled  AWVariant=Passthrough  PCopyVariant=Disabled  TRVariant=Disabled  FdbkBlocksVariant=Forward  IdealPFdbkVariant=Disabled  SatFdbkVariant=Disabled  DerivativeFilterVariant=ContFilter  NVariant=InternalParameters  NCopyVariant=Disabled  FilterICVariant=InternalICsFilter  IntegratorICVariant=InternalICs  ExternalResetVariant=Disabled  TRSumVariant=Passthrough  SumFdbkVariant=Disabled  SumVariant=Sum_PID  TsampFilterVariant=InternalTs  TsampNgainVariant=Passthrough  TsampIntegralVariant=Disabled_SignalSpec  ExternalSaturationOutDataTypeStr=Inherit: Same as second input
  Subsystem2 : Subsystem  Commented=on
  Sum1 : Sum  Commented=on  Inputs=|+-
  Switch1 : Switch  Commented=on  Criteria=u2 ~= 0  Threshold=1  SaturateOnIntegerOverflow=off  InputSameDT=off
  drive pulley velocity : Outport
  load velocity : Outport  Port=2
  load position : Outport  Port=3
  driven pulley Velocity : Outport  Port=4
  wires:
  Switch1/1 -> Sum1/1
  Sum1/1 -> PID Controller1/1
  V1/1 -> Switch1/2
  Subsystem2/2(load velocity) -> load velocity/1, Sum1/2  "Velocity"
  Constant3/1 -> Switch1/1
  Constant4/1 -> Switch1/3
  PID Controller1/1 -> Subsystem2/1(Voltage)
  Subsystem2/3(load position) -> load position/1
  Subsystem2/4(driven pulley Velocity) -> driven pulley Velocity/1
  Subsystem2/1(drive pulley velocity) -> drive pulley velocity/1

== system TopLevelModel/Belt3 ==
  V1 : Inport
  Constant3 : Constant  Commented=on  Value=0.2
  Constant4 : Constant  Commented=on  Value=0
  PID Controller1 : slpidlib/PID Controller  Commented=on  Controller=PID  Form=Parallel  TimeDomain=Continuous-time  UseExternalTs=off  SampleTime=-1  IntegratorMethod=Forward Euler  FilterMethod=Forward Euler  ControllerParametersSource=internal  P=29.8496571480823  I=152.933850283855  UseKiTs=off  D=-0.451147774638306  N=4.48716691500189  UseFilter=on  TunerSelectOption=Transfer Function Based (PID Tuner App)  InitialConditionSource=internal  InitialConditionForIntegrator=0  InitialConditionForFilter=0  DifferentiatorICPrevScaledInput=0  ExternalReset=none  TrackingMode=off  Kt=1  LimitOutput=off  SatLimitsSource=internal  UpperSaturationLimit=inf  LowerSaturationLimit=-inf  LinearizeAsGain=on  AntiWindupMode=none  Kb=1  LimitIntegrator=off  UpperIntegratorSaturationLimit=inf  LowerIntegratorSaturationLimit=-inf  POutMin=[]  POutMax=[]  IOutMin=[]  IOutMax=[]  DOutMin=[]  DOutMax=[]  NOutMin=[]  NOutMax=[]  SumOutMin=[]  SumOutMax=[]  SaturationOutMin=[]  SaturationOutMax=[]  PParamMin=[]  PParamMax=[]  IParamMin=[]  IParamMax=[]  DParamMin=[]  DParamMax=[]  NParamMin=[]  NParamMax=[]  KbParamMin=[]  KbParamMax=[]  KtParamMin=[]  KtParamMax=[]  KbOutMin=[]  KbOutMax=[]  KtOutMin=[]  KtOutMax=[]  IntegratorOutMin=[]  IntegratorOutMax=[]  FilterOutMin=[]  FilterOutMax=[]  SumI1OutMin=[]  SumI1OutMax=[]  SumI2OutMin=[]  SumI2OutMax=[]  SumI3OutMin=[]  SumI3OutMax=[]  SumI4OutMin=[]  SumI4OutMax=[]  SumDOutMin=[]  SumDOutMax=[]  DifferentiatorOutMin=[]  DifferentiatorOutMax=[]  FilterDiffOutCoefMin=[]  FilterDiffOutCoefMax=[]  ReciprocalOutMin=[]  ReciprocalOutMax=[]  SumDenOutMin=[]  SumDenOutMax=[]  SumNumOutMin=[]  SumNumOutMax=[]  DivideOutMin=[]  DivideOutMax=[]  UdiffTsProdOutMin=[]  UdiffTsProdOutMax=[]  NTsProdOutMin=[]  NTsProdOutMax=[]  UintegralTsProdOutMin=[]  UintegralTsProdOutMax=[]  UngainTsProdOutMin=[]  UngainTsProdOutMax=[]  ClampingZeroOutDataTypeStr=Inherit: Inherit via back propagation  ClampingZeroOutMin=[]  ClampingZeroOutMax=[]  FilterDenConstantOutDataTypeStr=Inherit: Inherit via back propagation  FilterDenConstantOutMin=[]  FilterDenConstantOutMax=[]  PCopyOutDataTypeStr=Inherit: Inherit via back propagation  PCopyOutMin=[]  PCopyOutMax=[]  NCopyOutDataTypeStr=Inherit: Inherit via back propagation  NCopyOutMin=[]  NCopyOutMax=[]  IntegratorContinuousStateAttributes=''  IntegratorStateMustResolveToSignalObject=off  IntegratorRTWStateStorageClass=Auto  FilterContinuousStateAttributes=''  FilterStateMustResolveToSignalObject=off  FilterRTWStateStorageClass=Auto  ParallelPVariant=InternalParameters  IdealPVariant=Disabled  IVariant=InternalParameters  DVariant=InternalParameters  IntegratorVariant=Continuous  SatVariant=Disabled  AWVariant=Passthrough  PCopyVariant=Disabled  TRVariant=Disabled  FdbkBlocksVariant=Forward  IdealPFdbkVariant=Disabled  SatFdbkVariant=Disabled  DerivativeFilterVariant=ContFilter  NVariant=InternalParameters  NCopyVariant=Disabled  FilterICVariant=InternalICsFilter  IntegratorICVariant=InternalICs  ExternalResetVariant=Disabled  TRSumVariant=Passthrough  SumFdbkVariant=Disabled  SumVariant=Sum_PID  TsampFilterVariant=InternalTs  TsampNgainVariant=Passthrough  TsampIntegralVariant=Disabled_SignalSpec  ExternalSaturationOutDataTypeStr=Inherit: Same as second input
  Subsystem2 : Subsystem  Commented=on
  Sum1 : Sum  Commented=on  Inputs=|+-
  Switch1 : Switch  Commented=on  Criteria=u2 ~= 0  Threshold=1  SaturateOnIntegerOverflow=off  InputSameDT=off
  drive pulley velocity : Outport
  load velocity : Outport  Port=2
  load position : Outport  Port=3
  driven pulley Velocity : Outport  Port=4
  wires:
  Switch1/1 -> Sum1/1
  Sum1/1 -> PID Controller1/1
  V1/1 -> Switch1/2
  Subsystem2/2(load velocity) -> load velocity/1, Sum1/2  "Velocity"
  Constant3/1 -> Switch1/1
  Constant4/1 -> Switch1/3
  PID Controller1/1 -> Subsystem2/1(Voltage)
  Subsystem2/3(load position) -> load position/1
  Subsystem2/4(driven pulley Velocity) -> driven pulley Velocity/1
  Subsystem2/1(drive pulley velocity) -> drive pulley velocity/1

== system TopLevelModel/Belt4 ==
  V1 : Inport
  Constant3 : Constant  Commented=on  Value=0.2
  Constant4 : Constant  Commented=on  Value=0
  PID Controller1 : slpidlib/PID Controller  Commented=on  Controller=PID  Form=Parallel  TimeDomain=Continuous-time  UseExternalTs=off  SampleTime=-1  IntegratorMethod=Forward Euler  FilterMethod=Forward Euler  ControllerParametersSource=internal  P=29.8496571480823  I=152.933850283855  UseKiTs=off  D=-0.451147774638306  N=4.48716691500189  UseFilter=on  TunerSelectOption=Transfer Function Based (PID Tuner App)  InitialConditionSource=internal  InitialConditionForIntegrator=0  InitialConditionForFilter=0  DifferentiatorICPrevScaledInput=0  ExternalReset=none  TrackingMode=off  Kt=1  LimitOutput=off  SatLimitsSource=internal  UpperSaturationLimit=inf  LowerSaturationLimit=-inf  LinearizeAsGain=on  AntiWindupMode=none  Kb=1  LimitIntegrator=off  UpperIntegratorSaturationLimit=inf  LowerIntegratorSaturationLimit=-inf  POutMin=[]  POutMax=[]  IOutMin=[]  IOutMax=[]  DOutMin=[]  DOutMax=[]  NOutMin=[]  NOutMax=[]  SumOutMin=[]  SumOutMax=[]  SaturationOutMin=[]  SaturationOutMax=[]  PParamMin=[]  PParamMax=[]  IParamMin=[]  IParamMax=[]  DParamMin=[]  DParamMax=[]  NParamMin=[]  NParamMax=[]  KbParamMin=[]  KbParamMax=[]  KtParamMin=[]  KtParamMax=[]  KbOutMin=[]  KbOutMax=[]  KtOutMin=[]  KtOutMax=[]  IntegratorOutMin=[]  IntegratorOutMax=[]  FilterOutMin=[]  FilterOutMax=[]  SumI1OutMin=[]  SumI1OutMax=[]  SumI2OutMin=[]  SumI2OutMax=[]  SumI3OutMin=[]  SumI3OutMax=[]  SumI4OutMin=[]  SumI4OutMax=[]  SumDOutMin=[]  SumDOutMax=[]  DifferentiatorOutMin=[]  DifferentiatorOutMax=[]  FilterDiffOutCoefMin=[]  FilterDiffOutCoefMax=[]  ReciprocalOutMin=[]  ReciprocalOutMax=[]  SumDenOutMin=[]  SumDenOutMax=[]  SumNumOutMin=[]  SumNumOutMax=[]  DivideOutMin=[]  DivideOutMax=[]  UdiffTsProdOutMin=[]  UdiffTsProdOutMax=[]  NTsProdOutMin=[]  NTsProdOutMax=[]  UintegralTsProdOutMin=[]  UintegralTsProdOutMax=[]  UngainTsProdOutMin=[]  UngainTsProdOutMax=[]  ClampingZeroOutDataTypeStr=Inherit: Inherit via back propagation  ClampingZeroOutMin=[]  ClampingZeroOutMax=[]  FilterDenConstantOutDataTypeStr=Inherit: Inherit via back propagation  FilterDenConstantOutMin=[]  FilterDenConstantOutMax=[]  PCopyOutDataTypeStr=Inherit: Inherit via back propagation  PCopyOutMin=[]  PCopyOutMax=[]  NCopyOutDataTypeStr=Inherit: Inherit via back propagation  NCopyOutMin=[]  NCopyOutMax=[]  IntegratorContinuousStateAttributes=''  IntegratorStateMustResolveToSignalObject=off  IntegratorRTWStateStorageClass=Auto  FilterContinuousStateAttributes=''  FilterStateMustResolveToSignalObject=off  FilterRTWStateStorageClass=Auto  ParallelPVariant=InternalParameters  IdealPVariant=Disabled  IVariant=InternalParameters  DVariant=InternalParameters  IntegratorVariant=Continuous  SatVariant=Disabled  AWVariant=Passthrough  PCopyVariant=Disabled  TRVariant=Disabled  FdbkBlocksVariant=Forward  IdealPFdbkVariant=Disabled  SatFdbkVariant=Disabled  DerivativeFilterVariant=ContFilter  NVariant=InternalParameters  NCopyVariant=Disabled  FilterICVariant=InternalICsFilter  IntegratorICVariant=InternalICs  ExternalResetVariant=Disabled  TRSumVariant=Passthrough  SumFdbkVariant=Disabled  SumVariant=Sum_PID  TsampFilterVariant=InternalTs  TsampNgainVariant=Passthrough  TsampIntegralVariant=Disabled_SignalSpec  ExternalSaturationOutDataTypeStr=Inherit: Same as second input
  Subsystem2 : Subsystem  Commented=on
  Sum1 : Sum  Commented=on  Inputs=|+-
  Switch1 : Switch  Commented=on  Criteria=u2 ~= 0  Threshold=1  SaturateOnIntegerOverflow=off  InputSameDT=off
  drive pulley velocity : Outport
  load velocity : Outport  Port=2
  load position : Outport  Port=3
  driven pulley Velocity : Outport  Port=4
  wires:
  Switch1/1 -> Sum1/1
  Sum1/1 -> PID Controller1/1
  V1/1 -> Switch1/2
  Subsystem2/2(load velocity) -> load velocity/1, Sum1/2  "Velocity"
  Constant3/1 -> Switch1/1
  Constant4/1 -> Switch1/3
  PID Controller1/1 -> Subsystem2/1(Voltage)
  Subsystem2/3(load position) -> load position/1
  Subsystem2/4(driven pulley Velocity) -> driven pulley Velocity/1
  Subsystem2/1(drive pulley velocity) -> drive pulley velocity/1

== system TopLevelModel/Belt5 ==
  V1 : Inport
  Constant3 : Constant  Commented=on  Value=0.2
  Constant4 : Constant  Commented=on  Value=0
  PID Controller1 : slpidlib/PID Controller  Commented=on  Controller=PID  Form=Parallel  TimeDomain=Continuous-time  UseExternalTs=off  SampleTime=-1  IntegratorMethod=Forward Euler  FilterMethod=Forward Euler  ControllerParametersSource=internal  P=29.8496571480823  I=152.933850283855  UseKiTs=off  D=-0.451147774638306  N=4.48716691500189  UseFilter=on  TunerSelectOption=Transfer Function Based (PID Tuner App)  InitialConditionSource=internal  InitialConditionForIntegrator=0  InitialConditionForFilter=0  DifferentiatorICPrevScaledInput=0  ExternalReset=none  TrackingMode=off  Kt=1  LimitOutput=off  SatLimitsSource=internal  UpperSaturationLimit=inf  LowerSaturationLimit=-inf  LinearizeAsGain=on  AntiWindupMode=none  Kb=1  LimitIntegrator=off  UpperIntegratorSaturationLimit=inf  LowerIntegratorSaturationLimit=-inf  POutMin=[]  POutMax=[]  IOutMin=[]  IOutMax=[]  DOutMin=[]  DOutMax=[]  NOutMin=[]  NOutMax=[]  SumOutMin=[]  SumOutMax=[]  SaturationOutMin=[]  SaturationOutMax=[]  PParamMin=[]  PParamMax=[]  IParamMin=[]  IParamMax=[]  DParamMin=[]  DParamMax=[]  NParamMin=[]  NParamMax=[]  KbParamMin=[]  KbParamMax=[]  KtParamMin=[]  KtParamMax=[]  KbOutMin=[]  KbOutMax=[]  KtOutMin=[]  KtOutMax=[]  IntegratorOutMin=[]  IntegratorOutMax=[]  FilterOutMin=[]  FilterOutMax=[]  SumI1OutMin=[]  SumI1OutMax=[]  SumI2OutMin=[]  SumI2OutMax=[]  SumI3OutMin=[]  SumI3OutMax=[]  SumI4OutMin=[]  SumI4OutMax=[]  SumDOutMin=[]  SumDOutMax=[]  DifferentiatorOutMin=[]  DifferentiatorOutMax=[]  FilterDiffOutCoefMin=[]  FilterDiffOutCoefMax=[]  ReciprocalOutMin=[]  ReciprocalOutMax=[]  SumDenOutMin=[]  SumDenOutMax=[]  SumNumOutMin=[]  SumNumOutMax=[]  DivideOutMin=[]  DivideOutMax=[]  UdiffTsProdOutMin=[]  UdiffTsProdOutMax=[]  NTsProdOutMin=[]  NTsProdOutMax=[]  UintegralTsProdOutMin=[]  UintegralTsProdOutMax=[]  UngainTsProdOutMin=[]  UngainTsProdOutMax=[]  ClampingZeroOutDataTypeStr=Inherit: Inherit via back propagation  ClampingZeroOutMin=[]  ClampingZeroOutMax=[]  FilterDenConstantOutDataTypeStr=Inherit: Inherit via back propagation  FilterDenConstantOutMin=[]  FilterDenConstantOutMax=[]  PCopyOutDataTypeStr=Inherit: Inherit via back propagation  PCopyOutMin=[]  PCopyOutMax=[]  NCopyOutDataTypeStr=Inherit: Inherit via back propagation  NCopyOutMin=[]  NCopyOutMax=[]  IntegratorContinuousStateAttributes=''  IntegratorStateMustResolveToSignalObject=off  IntegratorRTWStateStorageClass=Auto  FilterContinuousStateAttributes=''  FilterStateMustResolveToSignalObject=off  FilterRTWStateStorageClass=Auto  ParallelPVariant=InternalParameters  IdealPVariant=Disabled  IVariant=InternalParameters  DVariant=InternalParameters  IntegratorVariant=Continuous  SatVariant=Disabled  AWVariant=Passthrough  PCopyVariant=Disabled  TRVariant=Disabled  FdbkBlocksVariant=Forward  IdealPFdbkVariant=Disabled  SatFdbkVariant=Disabled  DerivativeFilterVariant=ContFilter  NVariant=InternalParameters  NCopyVariant=Disabled  FilterICVariant=InternalICsFilter  IntegratorICVariant=InternalICs  ExternalResetVariant=Disabled  TRSumVariant=Passthrough  SumFdbkVariant=Disabled  SumVariant=Sum_PID  TsampFilterVariant=InternalTs  TsampNgainVariant=Passthrough  TsampIntegralVariant=Disabled_SignalSpec  ExternalSaturationOutDataTypeStr=Inherit: Same as second input
  Subsystem2 : Subsystem  Commented=on
  Sum1 : Sum  Commented=on  Inputs=|+-
  Switch1 : Switch  Commented=on  Criteria=u2 ~= 0  Threshold=1  SaturateOnIntegerOverflow=off  InputSameDT=off
  drive pulley velocity : Outport
  load velocity : Outport  Port=2
  load position : Outport  Port=3
  driven pulley Velocity : Outport  Port=4
  wires:
  Switch1/1 -> Sum1/1
  Sum1/1 -> PID Controller1/1
  V1/1 -> Switch1/2
  Subsystem2/2(load velocity) -> load velocity/1, Sum1/2  "Velocity"
  Constant3/1 -> Switch1/1
  Constant4/1 -> Switch1/3
  PID Controller1/1 -> Subsystem2/1(Voltage)
  Subsystem2/3(load position) -> load position/1
  Subsystem2/4(driven pulley Velocity) -> driven pulley Velocity/1
  Subsystem2/1(drive pulley velocity) -> drive pulley velocity/1

== system TopLevelModel/Belt6 ==
  V1 : Inport
  Constant3 : Constant  Commented=on  Value=0.2
  Constant4 : Constant  Commented=on  Value=0
  PID Controller1 : slpidlib/PID Controller  Commented=on  Controller=PID  Form=Parallel  TimeDomain=Continuous-time  UseExternalTs=off  SampleTime=-1  IntegratorMethod=Forward Euler  FilterMethod=Forward Euler  ControllerParametersSource=internal  P=29.8496571480823  I=152.933850283855  UseKiTs=off  D=-0.451147774638306  N=4.48716691500189  UseFilter=on  TunerSelectOption=Transfer Function Based (PID Tuner App)  InitialConditionSource=internal  InitialConditionForIntegrator=0  InitialConditionForFilter=0  DifferentiatorICPrevScaledInput=0  ExternalReset=none  TrackingMode=off  Kt=1  LimitOutput=off  SatLimitsSource=internal  UpperSaturationLimit=inf  LowerSaturationLimit=-inf  LinearizeAsGain=on  AntiWindupMode=none  Kb=1  LimitIntegrator=off  UpperIntegratorSaturationLimit=inf  LowerIntegratorSaturationLimit=-inf  POutMin=[]  POutMax=[]  IOutMin=[]  IOutMax=[]  DOutMin=[]  DOutMax=[]  NOutMin=[]  NOutMax=[]  SumOutMin=[]  SumOutMax=[]  SaturationOutMin=[]  SaturationOutMax=[]  PParamMin=[]  PParamMax=[]  IParamMin=[]  IParamMax=[]  DParamMin=[]  DParamMax=[]  NParamMin=[]  NParamMax=[]  KbParamMin=[]  KbParamMax=[]  KtParamMin=[]  KtParamMax=[]  KbOutMin=[]  KbOutMax=[]  KtOutMin=[]  KtOutMax=[]  IntegratorOutMin=[]  IntegratorOutMax=[]  FilterOutMin=[]  FilterOutMax=[]  SumI1OutMin=[]  SumI1OutMax=[]  SumI2OutMin=[]  SumI2OutMax=[]  SumI3OutMin=[]  SumI3OutMax=[]  SumI4OutMin=[]  SumI4OutMax=[]  SumDOutMin=[]  SumDOutMax=[]  DifferentiatorOutMin=[]  DifferentiatorOutMax=[]  FilterDiffOutCoefMin=[]  FilterDiffOutCoefMax=[]  ReciprocalOutMin=[]  ReciprocalOutMax=[]  SumDenOutMin=[]  SumDenOutMax=[]  SumNumOutMin=[]  SumNumOutMax=[]  DivideOutMin=[]  DivideOutMax=[]  UdiffTsProdOutMin=[]  UdiffTsProdOutMax=[]  NTsProdOutMin=[]  NTsProdOutMax=[]  UintegralTsProdOutMin=[]  UintegralTsProdOutMax=[]  UngainTsProdOutMin=[]  UngainTsProdOutMax=[]  ClampingZeroOutDataTypeStr=Inherit: Inherit via back propagation  ClampingZeroOutMin=[]  ClampingZeroOutMax=[]  FilterDenConstantOutDataTypeStr=Inherit: Inherit via back propagation  FilterDenConstantOutMin=[]  FilterDenConstantOutMax=[]  PCopyOutDataTypeStr=Inherit: Inherit via back propagation  PCopyOutMin=[]  PCopyOutMax=[]  NCopyOutDataTypeStr=Inherit: Inherit via back propagation  NCopyOutMin=[]  NCopyOutMax=[]  IntegratorContinuousStateAttributes=''  IntegratorStateMustResolveToSignalObject=off  IntegratorRTWStateStorageClass=Auto  FilterContinuousStateAttributes=''  FilterStateMustResolveToSignalObject=off  FilterRTWStateStorageClass=Auto  ParallelPVariant=InternalParameters  IdealPVariant=Disabled  IVariant=InternalParameters  DVariant=InternalParameters  IntegratorVariant=Continuous  SatVariant=Disabled  AWVariant=Passthrough  PCopyVariant=Disabled  TRVariant=Disabled  FdbkBlocksVariant=Forward  IdealPFdbkVariant=Disabled  SatFdbkVariant=Disabled  DerivativeFilterVariant=ContFilter  NVariant=InternalParameters  NCopyVariant=Disabled  FilterICVariant=InternalICsFilter  IntegratorICVariant=InternalICs  ExternalResetVariant=Disabled  TRSumVariant=Passthrough  SumFdbkVariant=Disabled  SumVariant=Sum_PID  TsampFilterVariant=InternalTs  TsampNgainVariant=Passthrough  TsampIntegralVariant=Disabled_SignalSpec  ExternalSaturationOutDataTypeStr=Inherit: Same as second input
  Subsystem2 : Subsystem  Commented=on
  Sum1 : Sum  Commented=on  Inputs=|+-
  Switch1 : Switch  Commented=on  Criteria=u2 ~= 0  Threshold=1  SaturateOnIntegerOverflow=off  InputSameDT=off
  drive pulley velocity : Outport
  load velocity : Outport  Port=2
  load position : Outport  Port=3
  driven pulley Velocity : Outport  Port=4
  wires:
  Switch1/1 -> Sum1/1
  Sum1/1 -> PID Controller1/1
  V1/1 -> Switch1/2
  Subsystem2/2(load velocity) -> load velocity/1, Sum1/2  "Velocity"
  Constant3/1 -> Switch1/1
  Constant4/1 -> Switch1/3
  PID Controller1/1 -> Subsystem2/1(Voltage)
  Subsystem2/3(load position) -> load position/1
  Subsystem2/4(driven pulley Velocity) -> driven pulley Velocity/1
  Subsystem2/1(drive pulley velocity) -> drive pulley velocity/1
